simulink subsystem "Sensormodel"  (R2024b)
settings: Solver=VariableStepAuto  StartTime=0.0  StopTime=10.0  RelTol=1e-3
undefined symbols (not defined in the file): accel, gyro
libraries: simulink x2
settings Model: Creator=Marij  LastModifiedBy=marijn

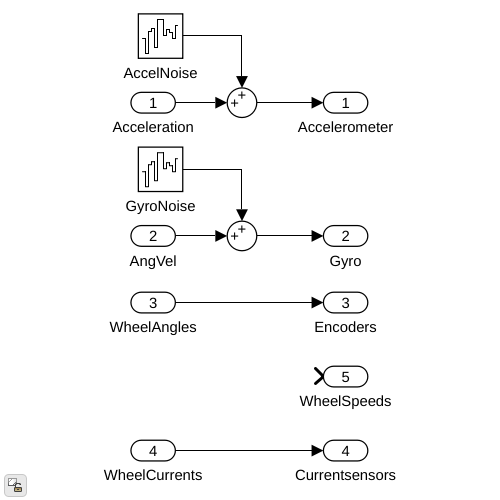
[thumbnail: Simulink's stored preview of the top-level diagram]
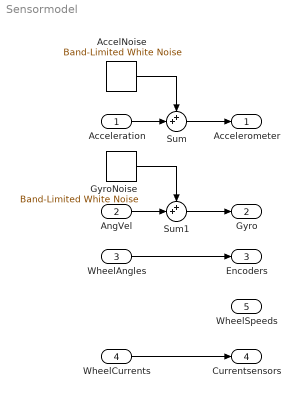
== system Sensormodel ==
  Acceleration : Inport  Unit=m/s^2  PortDimensions=2
  AngVel : Inport  Port=2  Unit=rad/s  PortDimensions=1
  WheelAngles : Inport  Port=3  Unit=rad  PortDimensions=4
  WheelCurrents : Inport  Port=4  Unit=A  PortDimensions=4
  AccelNoise : simulink/Sources/Band-Limited White Noise  Cov=[accel.noise, accel.noise]  Ts=0.01  seed=[23341]
  GyroNoise : simulink/Sources/Band-Limited White Noise  Cov=[gyro.noise]  Ts=0.01  seed=[23341]
  Sum : Sum  Inputs=++|
  Sum1 : Sum  Inputs=++|
  Accelerometer : Outport  Unit=m/s^2  PortDimensions=2
  Gyro : Outport  Port=2  Unit=rad/s  PortDimensions=1
  Encoders : Outport  Port=3  Unit=rad  PortDimensions=4
  Currentsensors : Outport  Port=4  Unit=A  PortDimensions=4
  WheelSpeeds : Outport  Port=5  Unit=rad/s  PortDimensions=4
  wires:
  AccelNoise/1 -> Sum/1
  Sum/1 -> Accelerometer/1
  Acceleration/1 -> Sum/2
  Sum1/1 -> Gyro/1
  WheelCurrents/1 -> Currentsensors/1
  GyroNoise/1 -> Sum1/1
  AngVel/1 -> Sum1/2
  WheelAngles/1 -> Encoders/1
